simulink model "building3s"  (R2017a)
settings: Solver=ode14x  StartTime=0.0  StopTime=5  FixedStep=0.01  RelTol=1e-3
InitFcn:
  | kpmin=100;
  | kpmax=700;
  | kdmin=50;
  | kdmax=400;
values from neighbouring files (symbols this model uses):
  a = 175/98.3    (= 1.78026449644)    [Untitled.m]
  b = 50/98.3    (= 0.508646998983)    [Untitled.m]
  c = 1200000/98.3    (= 12207.5279756)    [Untitled.m]
  d = 684000/98.3    (= 6958.29094608)    [Untitled.m]
  e = 100/98.3    (= 1.01729399797)    [Untitled.m]
  f = 1370000/98.3    (= 13936.9277721)    [Untitled.m]
  jerm = 98.3    [Untitled.m]
  kkd = 253.2802    [Untitled.m]
  kki = 100    [Untitled.m]
  kkp = 570    [Untitled.m]
libraries: fuzblock x2, simulink x1
settings Model: Creator=Amir  LastModifiedBy=ASUS

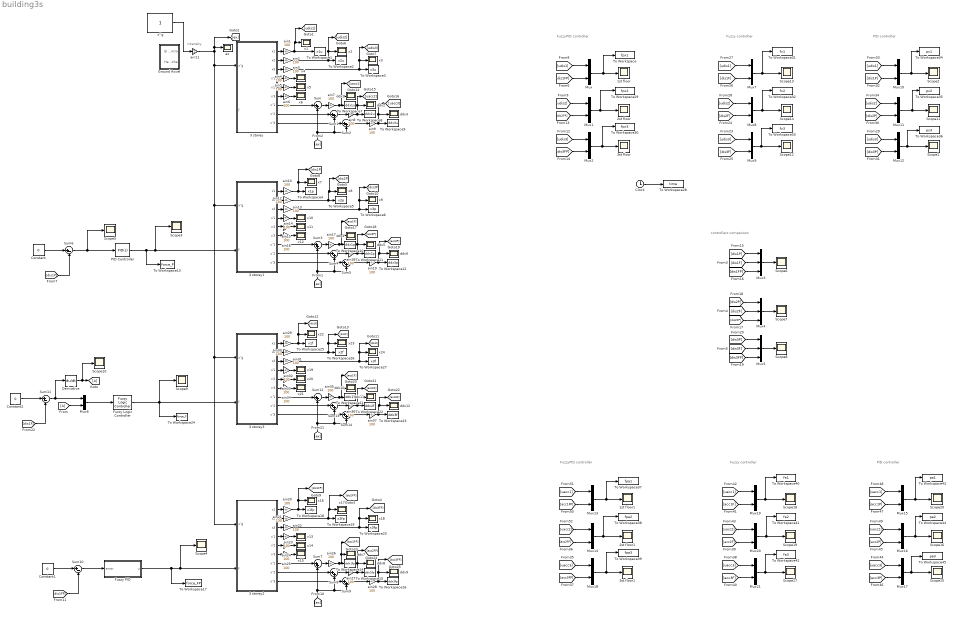
== system building3s ==
  note: controllers comparison
  note: Fuzzy controller
  note: FuzzyPID controller
  note: intensity
  note: PID controller
  note: Fuzzy controller
  note: FuzzyPID controller
  note: PID controller
  1st floor : Scope
  1st floor1 : Scope
  2st floor : Scope
  2st floor1 : Scope
  3 storey : Subsystem
  3 storey1 : Subsystem
  3 storey2 : Subsystem
  3 storey3 : Subsystem
  3st floor : Scope
  3st floor1 : Scope
  Clock : Clock
  Constant : Constant  Value=0
  Constant1 : Constant  Value=0
  Constant2 : Constant  Value=0
  Derivative : Derivative
  Fuzzy Logic Controller : fuzblock/Fuzzy Logic  Controller  fis=fuzz1
  Fuzzy PID : Subsystem
  Ground Accel : Subsystem
  Mux{,1..2,6..21} (19 alike) : Mux  Inputs=2
  Mux3 : Mux  Inputs=3
  Mux4 : Mux  Inputs=3
  Mux5 : Mux  Inputs=3
  PID Controller : simulink/Continuous/PID Controller  Controller=PID  TimeDomain=Continuous-time  SampleTime=-1  IntegratorMethod=Forward Euler  FilterMethod=Forward Euler  Form=Parallel  UseFilter=on  ControllerParametersSource=internal  P=kkp  I=kki  D=kkd  N=100  InitialConditionSource=internal  InitialConditionForIntegrator=0  InitialConditionForFilter=0  ExternalReset=none  LimitOutput=off  UpperSaturationLimit=inf  LowerSaturationLimit=-inf  LinearizeAsGain=on  AntiWindupMode=none  Kb=1  TrackingMode=off  Kt=1  PParamMin=[]  PParamMax=[]  IParamMin=[]  IParamMax=[]  DParamMin=[]  DParamMax=[]  NParamMin=[]  NParamMax=[]  KbParamMin=[]  KbParamMax=[]  KtParamMin=[]  KtParamMax=[]  POutMin=[]  POutMax=[]  IOutMin=[]  IOutMax=[]  DOutMin=[]  DOutMax=[]  NOutMin=[]  NOutMax=[]  KbOutMin=[]  KbOutMax=[]  KtOutMin=[]  KtOutMax=[]  IntegratorOutMin=[]  IntegratorOutMax=[]  FilterOutMin=[]  FilterOutMax=[]  SumOutMin=[]  SumOutMax=[]  SumI1OutMin=[]  SumI1OutMax=[]  SumI2OutMin=[]  SumI2OutMax=[]  SumI3OutMin=[]  SumI3OutMax=[]  SumDOutMin=[]  SumDOutMax=[]  SaturationOutMin=[]  SaturationOutMax=[]  IntegratorContinuousStateAttributes=''  IntegratorStateMustResolveToSignalObject=off  IntegratorRTWStateStorageClass=Auto  FilterContinuousStateAttributes=''  FilterStateMustResolveToSignalObject=off  FilterRTWStateStorageClass=Auto  DifferentiatorICPrevScaledInput=0  DifferentiatorOutMin=[]  DifferentiatorOutMax=[]  InitialConditionSetting=State (most efficient)
  Scope{1..20} (20 alike) : Scope
  Sum{,1..5,7..9,12..14} (12 alike) : Sum  Inputs=|++
  Sum10 : Sum  Inputs=|+-
  Sum11 : Sum  Inputs=|+-
  Sum6 : Sum  Inputs=|+-
  To Workspace : ToWorkspace  VariableName=fpx1  SampleTime=-1
  To Workspace1 : ToWorkspace  VariableName=x1u  SampleTime=-1
  To Workspace10 : ToWorkspace  VariableName=ddx1p  SampleTime=-1
  To Workspace11 : ToWorkspace  VariableName=ddx2p  SampleTime=-1
  To Workspace12 : ToWorkspace  VariableName=ddx3p  SampleTime=-1
  To Workspace13 : ToWorkspace  VariableName=force_P  SampleTime=-1
  To Workspace14 : ToWorkspace  VariableName=ddx1fp  SampleTime=-1
  To Workspace15 : ToWorkspace  VariableName=ddx2fp  SampleTime=-1
  To Workspace16 : ToWorkspace  VariableName=ddx3fp  SampleTime=-1
  To Workspace17 : ToWorkspace  VariableName=force_FP  SampleTime=-1
  To Workspace18 : ToWorkspace  VariableName=x1fp  SampleTime=-1
  To Workspace19 : ToWorkspace  VariableName=x2fp  SampleTime=-1
  To Workspace2 : ToWorkspace  VariableName=x2u  SampleTime=-1
  To Workspace20 : ToWorkspace  VariableName=x3fp  SampleTime=-1
  To Workspace21 : ToWorkspace  VariableName=ddx1f  SampleTime=-1
  To Workspace22 : ToWorkspace  VariableName=ddx2f  SampleTime=-1
  To Workspace23 : ToWorkspace  VariableName=ddx3f  SampleTime=-1
  To Workspace24 : ToWorkspace  VariableName=force_F  SampleTime=-1
  To Workspace25 : ToWorkspace  VariableName=x1f  SampleTime=-1
  To Workspace26 : ToWorkspace  VariableName=x2f  SampleTime=-1
  To Workspace27 : ToWorkspace  VariableName=x3f  SampleTime=-1
  To Workspace28 : ToWorkspace  VariableName=time  SampleTime=-1
  To Workspace29 : ToWorkspace  VariableName=fpx2  SampleTime=-1
  To Workspace3 : ToWorkspace  VariableName=x3u  SampleTime=-1
  To Workspace30 : ToWorkspace  VariableName=fpx3  SampleTime=-1
  To Workspace31 : ToWorkspace  VariableName=fx1  SampleTime=-1
  To Workspace32 : ToWorkspace  VariableName=fx2  SampleTime=-1
  To Workspace33 : ToWorkspace  VariableName=fx3  SampleTime=-1
  To Workspace34 : ToWorkspace  VariableName=px1  SampleTime=-1
  To Workspace35 : ToWorkspace  VariableName=px2  SampleTime=-1
  To Workspace36 : ToWorkspace  VariableName=px3  SampleTime=-1
  To Workspace37 : ToWorkspace  VariableName=fpa1  SampleTime=-1
  To Workspace38 : ToWorkspace  VariableName=fpa2  SampleTime=-1
  To Workspace39 : ToWorkspace  VariableName=fpa3  SampleTime=-1
  To Workspace4 : ToWorkspace  VariableName=x1p  SampleTime=-1
  To Workspace40 : ToWorkspace  VariableName=fa1  SampleTime=-1
  To Workspace41 : ToWorkspace  VariableName=fa2  SampleTime=-1
  To Workspace42 : ToWorkspace  VariableName=fa3  SampleTime=-1
  To Workspace43 : ToWorkspace  VariableName=pa1  SampleTime=-1
  To Workspace44 : ToWorkspace  VariableName=pa2  SampleTime=-1
  To Workspace45 : ToWorkspace  VariableName=pa3  SampleTime=-1
  To Workspace5 : ToWorkspace  VariableName=x2p  SampleTime=-1
  To Workspace6 : ToWorkspace  VariableName=x3p  SampleTime=-1
  To Workspace7 : ToWorkspace  VariableName=ddx1u  SampleTime=-1
  To Workspace8 : ToWorkspace  VariableName=ddx2u  SampleTime=-1
  To Workspace9 : ToWorkspace  VariableName=ddx3u  SampleTime=-1
  ain{1..10,12..37} (36 alike) : Gain  Gain=100
  ain11 : Gain
  ddx{1..12} (12 alike) : Scope
  ex : Scope
  x''g : Constant
  x{1..24} (24 alike) : Scope
  wires:
  ain3/1 -> To Workspace3/1, [udis3], x3/1
  3 storey/8(x''2) -> Sum1/1
  Sum/1 -> ain7/1
  [ex] -> Sum/2, Sum1/2, Sum2/2
  3 storey/5(x'2) -> ain5/1
  Sum2/1 -> ain9/1
  3 storey/7(x''1) -> Sum/1
  3 storey/9(x''3) -> Sum2/1
  ain9/1 -> To Workspace9/1, [uacc3], ddx3/1
  Sum1/1 -> ain8/1
  ain4/1 -> x4/1
  3 storey/6(x'3) -> ain6/1
  3 storey/4(x'1) -> ain4/1
  ain2/1 -> To Workspace2/1, [udis2], x2/1
  ain5/1 -> x5/1
  ain6/1 -> x6/1
  3 storey/3(x3) -> ain3/1
  ain7/1 -> To Workspace7/1, [uacc1], ddx1/1
  3 storey/2(x2) -> ain2/1
  ain1/1 -> To Workspace1/1, [udis1], x1/1
  ain11/1 -> 3 storey1/1(x''g), 3 storey2/1(x''g), 3 storey3/1(x''g), 3 storey/1(x''g), [ex], ex/1
  ain8/1 -> To Workspace8/1, ddx2/1, [uacc2]
  3 storey/1(x1) -> ain1/1
  x''g/1 -> ain11/1
  ain25/1 -> x15/1
  Sum7/1 -> ain26/1
  Sum10/1 -> Fuzzy PID/1(error)
  Constant1/1 -> Sum10/1
  3 storey2/8(x''2) -> Sum8/1
  [dis1FP] -> Sum10/2
  3 storey2/5(x'2) -> ain24/1
  Fuzzy PID/1(u) -> To Workspace17/1, Scope4/1, 3 storey2/2(f)
  ain22/1 -> [dis3FP], x18/1, To Workspace20/1
  3 storey2/2(x2) -> ain21/1
  [ex] -> Sum9/2, Sum8/2, Sum7/2
  Sum9/1 -> ain28/1
  3 storey2/3(x3) -> ain22/1
  ain26/1 -> [acc1FP], ddx7/1, To Workspace14/1
  ain28/1 -> [acc3FP], ddx9/1, To Workspace16/1
  ain20/1 -> [dis1FP], x16/1, To Workspace18/1
  ain21/1 -> [dis2FP], x17/1, To Workspace19/1
  Sum8/1 -> ain27/1
  3 storey2/6(x'3) -> ain25/1
  ain24/1 -> x14/1
  3 storey2/7(x''1) -> Sum7/1
  3 storey2/4(x'1) -> ain23/1
  3 storey2/1(x1) -> ain20/1
  3 storey2/9(x''3) -> Sum9/1
  ain23/1 -> x13/1
  ain27/1 -> [acc2FP], ddx8/1, To Workspace15/1
  3 storey1/8(x''2) -> Sum4/1
  ain14/1 -> x10/1
  3 storey1/1(x1) -> ain10/1
  ain10/1 -> [dis1P], x7/1, To Workspace4/1
  Sum3/1 -> ain17/1
  ain12/1 -> [dis2P], x8/1, To Workspace5/1
  ain19/1 -> [acc3P], ddx6/1, To Workspace12/1
  3 storey1/4(x'1) -> ain14/1
  ain17/1 -> [acc1P], ddx4/1, To Workspace10/1
  PID Controller/1 -> To Workspace13/1, Scope3/1, 3 storey1/2(f)
  Sum4/1 -> ain18/1
  ain18/1 -> [acc2P], ddx5/1, To Workspace11/1
  [ex] -> Sum5/2, Sum4/2, Sum3/2
  Sum5/1 -> ain19/1
  [dis1P] -> Sum6/2
  3 storey1/2(x2) -> ain12/1
  ain15/1 -> x11/1
  3 storey1/7(x''1) -> Sum3/1
  Constant/1 -> Sum6/1
  ain16/1 -> x12/1
  3 storey1/9(x''3) -> Sum5/1
  3 storey1/5(x'2) -> ain15/1
  ain13/1 -> [dis3P], x9/1, To Workspace6/1
  3 storey1/3(x3) -> ain13/1
  3 storey1/6(x'3) -> ain16/1
  Sum6/1 -> Scope5/1, PID Controller/1
  Mux5/1 -> Scope8/1
  Mux4/1 -> Scope7/1
  Mux3/1 -> Scope6/1
  [dis1FP] -> Mux3/3
  [dis1P] -> Mux3/1
  [dis2FP] -> Mux4/3
  [dis2P] -> Mux4/1
  [dis3P] -> Mux5/1
  [dis3FP] -> Mux5/3
  3 storey3/5(x'2) -> ain33/1
  ain36/1 -> ddx11/1, [acc2F], To Workspace22/1
  3 storey3/9(x''3) -> Sum14/1
  Constant2/1 -> Sum11/1
  ain30/1 -> [dis2F], x23/1, To Workspace26/1
  Derivative/1 -> Scope10/1, [A]
  [A] -> Mux6/2
  [ex] -> Sum14/2, Sum13/2, Sum12/2
  ain32/1 -> x19/1
  ain33/1 -> x20/1
  ain31/1 -> [dis3F], x24/1, To Workspace27/1
  Fuzzy Logic Controller/1 -> Scope9/1, 3 storey3/2(f), To Workspace24/1
  3 storey3/8(x''2) -> Sum13/1
  ain35/1 -> [acc1F], ddx10/1, To Workspace21/1
  Sum11/1 -> Derivative/1, Mux6/1
  ain34/1 -> x21/1
  Mux6/1 -> Fuzzy Logic Controller/1
  3 storey3/1(x1) -> ain29/1
  3 storey3/7(x''1) -> Sum12/1
  3 storey3/4(x'1) -> ain32/1
  3 storey3/3(x3) -> ain31/1
  Sum14/1 -> ain37/1
  3 storey3/2(x2) -> ain30/1
  ain37/1 -> [acc3F], ddx12/1, To Workspace23/1
  Sum13/1 -> ain36/1
  3 storey3/6(x'3) -> ain34/1
  [dis1F] -> Sum11/2
  Sum12/1 -> ain35/1
  ain29/1 -> [dis1F], x22/1, To Workspace25/1
  [dis2F] -> Mux4/2
  [dis1F] -> Mux3/2
  [dis3F] -> Mux5/2
  Mux1/1 -> To Workspace29/1, 2st floor/1
  Mux/1 -> To Workspace/1, 1st floor/1
  Mux2/1 -> To Workspace30/1, 3st floor/1
  [udis3] -> Mux2/1
  [udis2] -> Mux1/1
  [dis3FP] -> Mux2/2
  [dis2FP] -> Mux1/2
  [dis1FP] -> Mux/2
  [udis1] -> Mux/1
  [udis3] -> Mux9/1
  [dis1F] -> Mux7/2
  [dis2F] -> Mux8/2
  [udis1] -> Mux7/1
  Mux8/1 -> To Workspace32/1, Scope14/1
  [dis3F] -> Mux9/2
  Mux7/1 -> To Workspace31/1, Scope13/1
  Mux9/1 -> To Workspace33/1, Scope12/1
  [udis2] -> Mux8/1
  Mux12/1 -> To Workspace36/1, Scope1/1
  Mux10/1 -> To Workspace34/1, Scope2/1
  [udis3] -> Mux12/1
  [udis2] -> Mux11/1
  [udis1] -> Mux10/1
  Mux11/1 -> To Workspace35/1, Scope11/1
  [dis1P] -> Mux10/2
  [dis3P] -> Mux12/2
  [dis2P] -> Mux11/2
  Clock/1 -> To Workspace28/1
  [acc2P] -> Mux16/2
  [acc3P] -> Mux17/2
  [acc1P] -> Mux15/2
  Mux16/1 -> Scope16/1, To Workspace44/1
  [uacc1] -> Mux15/1
  [uacc2] -> Mux16/1
  [uacc3] -> Mux17/1
  Mux15/1 -> Scope20/1, To Workspace43/1
  Mux17/1 -> Scope15/1, To Workspace45/1
  [uacc2] -> Mux20/1
  Mux21/1 -> Scope17/1, To Workspace42/1
  Mux19/1 -> Scope18/1, To Workspace40/1
  [acc3F] -> Mux21/2
  Mux20/1 -> Scope19/1, To Workspace41/1
  [uacc1] -> Mux19/1
  [acc2F] -> Mux20/2
  [acc1F] -> Mux19/2
  [uacc3] -> Mux21/1
  [uacc1] -> Mux13/1
  [acc1FP] -> Mux13/2
  [acc2FP] -> Mux14/2
  [acc3FP] -> Mux18/2
  [uacc2] -> Mux14/1
  [uacc3] -> Mux18/1
  Mux18/1 -> 3st floor1/1, To Workspace39/1
  Mux13/1 -> 1st floor1/1, To Workspace37/1
  Mux14/1 -> 2st floor1/1, To Workspace38/1

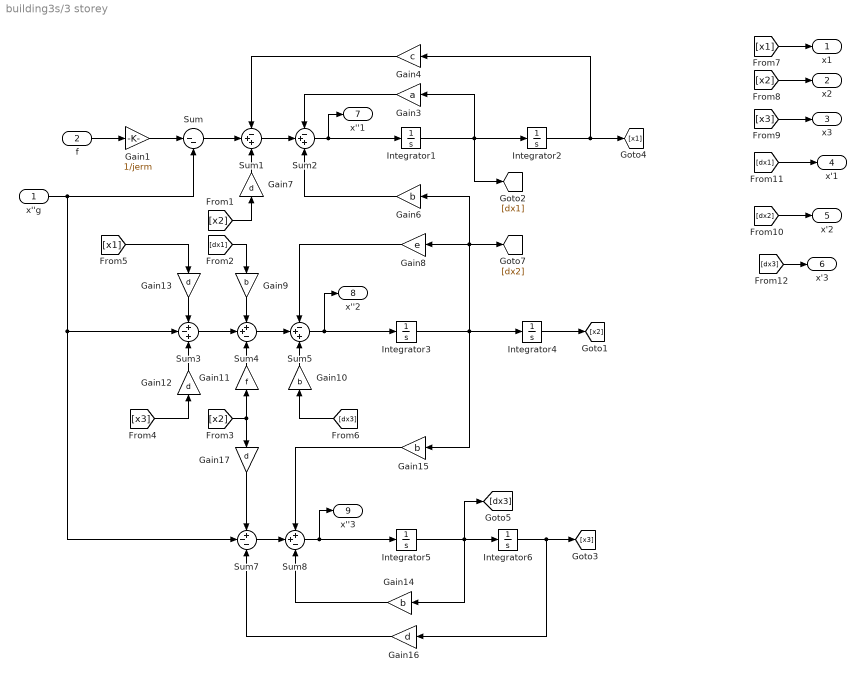
== system building3s/3 storey ==
  x''g : Inport
  f : Inport  Port=2
  Gain1 : Gain  Gain=1/jerm
  Gain{6,9..10,14..15} (5 alike) : Gain  Gain=b
  Gain11 : Gain  Gain=f
  Gain{7,12..13,16..17} (5 alike) : Gain  Gain=d
  Gain3 : Gain  Gain=a
  Gain4 : Gain  Gain=c
  Gain8 : Gain  Gain=e
  Integrator{1..6} (6 alike) : Integrator
  Sum : Sum  Inputs=|--
  Sum1 : Sum  Inputs=-++
  Sum2 : Sum  Inputs=-++
  Sum3 : Sum  Inputs=+-+
  Sum4 : Sum  Inputs=++-
  Sum5 : Sum  Inputs=-++
  Sum7 : Sum  Inputs=+--
  Sum8 : Sum  Inputs=++-
  x1 : Outport
  x2 : Outport  Port=2
  x3 : Outport  Port=3
  x'1 : Outport  Port=4
  x'2 : Outport  Port=5
  x'3 : Outport  Port=6
  x''1 : Outport  Port=7
  x''2 : Outport  Port=8
  x''3 : Outport  Port=9
  wires:
  Sum/1 -> Sum1/2
  Sum2/1 -> Integrator1/1, x''1/1
  Integrator1/1 -> Integrator2/1, Gain3/1, [dx1]
  f/1 -> Gain1/1
  Gain1/1 -> Sum/1
  Sum1/1 -> Sum2/2
  Sum3/1 -> Sum4/2
  Sum5/1 -> Integrator3/1, x''2/1
  Integrator3/1 -> Integrator4/1, Gain8/1, [dx2], Gain6/1, Gain15/1
  Sum4/1 -> Sum5/2
  Sum8/1 -> Integrator5/1, x''3/1
  Integrator5/1 -> Integrator6/1, Gain14/1, [dx3]
  Sum7/1 -> Sum8/2
  Gain3/1 -> Sum2/1
  Integrator2/1 -> Gain4/1, [x1]
  Gain4/1 -> Sum1/1
  Gain6/1 -> Sum2/3
  Integrator4/1 -> [x2]
  [x2] -> Gain7/1
  Gain7/1 -> Sum1/3
  x''g/1 -> Sum/2, Sum3/2, Sum7/2
  Gain8/1 -> Sum5/1
  [dx1] -> Gain9/1
  Gain9/1 -> Sum4/1
  [x2] -> Gain11/1, Gain17/1
  Gain11/1 -> Sum4/3
  Integrator6/1 -> [x3], Gain16/1
  [x3] -> Gain12/1
  Gain12/1 -> Sum3/3
  [x1] -> Gain13/1
  Gain13/1 -> Sum3/1
  Gain14/1 -> Sum8/3
  Gain16/1 -> Sum7/3
  [dx3] -> Gain10/1
  Gain10/1 -> Sum5/3
  [x1] -> x1/1
  [x2] -> x2/1
  [x3] -> x3/1
  [dx1] -> x'1/1
  [dx2] -> x'2/1
  [dx3] -> x'3/1
  Gain17/1 -> Sum7/1
  Gain15/1 -> Sum8/1

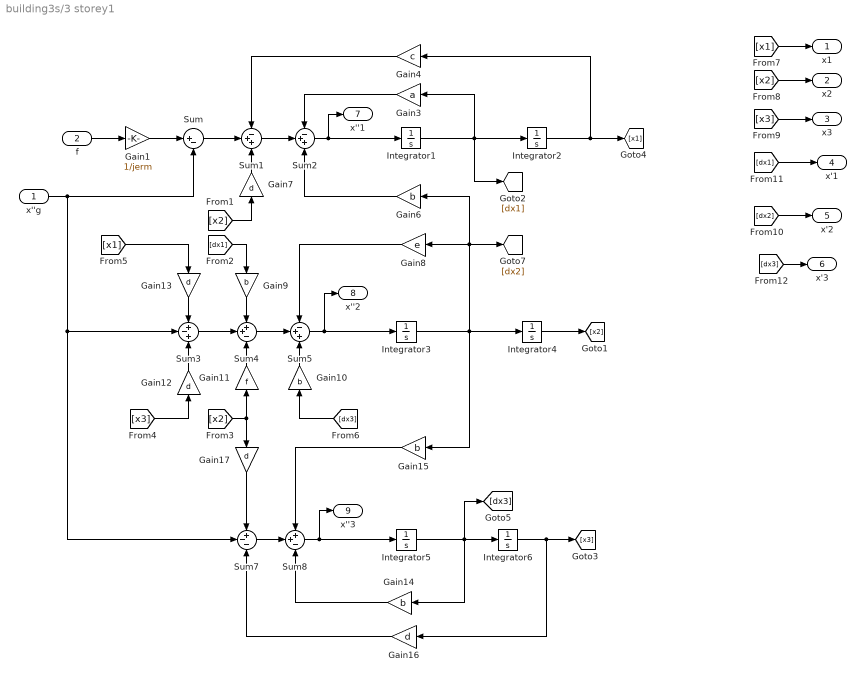
== system building3s/3 storey1 ==
  x''g : Inport
  f : Inport  Port=2
  Gain1 : Gain  Gain=1/jerm
  Gain{6,9..10,14..15} (5 alike) : Gain  Gain=b
  Gain11 : Gain  Gain=f
  Gain{7,12..13,16..17} (5 alike) : Gain  Gain=d
  Gain3 : Gain  Gain=a
  Gain4 : Gain  Gain=c
  Gain8 : Gain  Gain=e
  Integrator{1..6} (6 alike) : Integrator
  Sum : Sum  Inputs=|+-
  Sum1 : Sum  Inputs=-++
  Sum2 : Sum  Inputs=-++
  Sum3 : Sum  Inputs=+-+
  Sum4 : Sum  Inputs=++-
  Sum5 : Sum  Inputs=-++
  Sum7 : Sum  Inputs=+--
  Sum8 : Sum  Inputs=++-
  x1 : Outport
  x2 : Outport  Port=2
  x3 : Outport  Port=3
  x'1 : Outport  Port=4
  x'2 : Outport  Port=5
  x'3 : Outport  Port=6
  x''1 : Outport  Port=7
  x''2 : Outport  Port=8
  x''3 : Outport  Port=9
  wires:
  Gain15/1 -> Sum8/1
  Gain17/1 -> Sum7/1
  [dx3] -> x'3/1
  [dx2] -> x'2/1
  [dx1] -> x'1/1
  [x3] -> x3/1
  [x2] -> x2/1
  [x1] -> x1/1
  Gain10/1 -> Sum5/3
  [dx3] -> Gain10/1
  Gain16/1 -> Sum7/3
  Gain14/1 -> Sum8/3
  Gain13/1 -> Sum3/1
  [x1] -> Gain13/1
  Gain12/1 -> Sum3/3
  [x3] -> Gain12/1
  Integrator6/1 -> Gain16/1, [x3]
  Gain11/1 -> Sum4/3
  [x2] -> Gain17/1, Gain11/1
  Gain9/1 -> Sum4/1
  [dx1] -> Gain9/1
  Gain8/1 -> Sum5/1
  x''g/1 -> Sum7/2, Sum3/2, Sum/2
  Gain7/1 -> Sum1/3
  [x2] -> Gain7/1
  Integrator4/1 -> [x2]
  Gain6/1 -> Sum2/3
  Gain4/1 -> Sum1/1
  Integrator2/1 -> [x1], Gain4/1
  Gain3/1 -> Sum2/1
  Sum7/1 -> Sum8/2
  Integrator5/1 -> [dx3], Gain14/1, Integrator6/1
  Sum8/1 -> x''3/1, Integrator5/1
  Sum4/1 -> Sum5/2
  Integrator3/1 -> Gain15/1, Gain6/1, [dx2], Gain8/1, Integrator4/1
  Sum5/1 -> x''2/1, Integrator3/1
  Sum3/1 -> Sum4/2
  Sum1/1 -> Sum2/2
  Gain1/1 -> Sum/1
  f/1 -> Gain1/1
  Integrator1/1 -> [dx1], Gain3/1, Integrator2/1
  Sum2/1 -> x''1/1, Integrator1/1
  Sum/1 -> Sum1/2

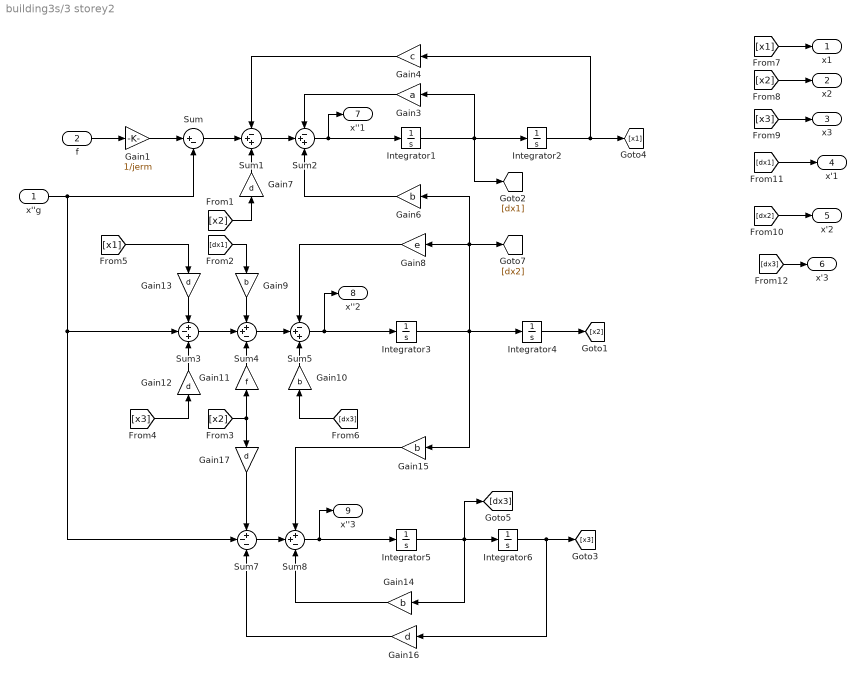
== system building3s/3 storey2 ==
  x''g : Inport
  f : Inport  Port=2
  Gain1 : Gain  Gain=1/jerm
  Gain{6,9..10,14..15} (5 alike) : Gain  Gain=b
  Gain11 : Gain  Gain=f
  Gain{7,12..13,16..17} (5 alike) : Gain  Gain=d
  Gain3 : Gain  Gain=a
  Gain4 : Gain  Gain=c
  Gain8 : Gain  Gain=e
  Integrator{1..6} (6 alike) : Integrator
  Sum : Sum  Inputs=|+-
  Sum1 : Sum  Inputs=-++
  Sum2 : Sum  Inputs=-++
  Sum3 : Sum  Inputs=+-+
  Sum4 : Sum  Inputs=++-
  Sum5 : Sum  Inputs=-++
  Sum7 : Sum  Inputs=+--
  Sum8 : Sum  Inputs=++-
  x1 : Outport
  x2 : Outport  Port=2
  x3 : Outport  Port=3
  x'1 : Outport  Port=4
  x'2 : Outport  Port=5
  x'3 : Outport  Port=6
  x''1 : Outport  Port=7
  x''2 : Outport  Port=8
  x''3 : Outport  Port=9
  wires:
  Gain15/1 -> Sum8/1
  Gain17/1 -> Sum7/1
  [dx3] -> x'3/1
  [dx2] -> x'2/1
  [dx1] -> x'1/1
  [x3] -> x3/1
  [x2] -> x2/1
  [x1] -> x1/1
  Gain10/1 -> Sum5/3
  [dx3] -> Gain10/1
  Gain16/1 -> Sum7/3
  Gain14/1 -> Sum8/3
  Gain13/1 -> Sum3/1
  [x1] -> Gain13/1
  Gain12/1 -> Sum3/3
  [x3] -> Gain12/1
  Integrator6/1 -> Gain16/1, [x3]
  Gain11/1 -> Sum4/3
  [x2] -> Gain17/1, Gain11/1
  Gain9/1 -> Sum4/1
  [dx1] -> Gain9/1
  Gain8/1 -> Sum5/1
  x''g/1 -> Sum7/2, Sum3/2, Sum/2
  Gain7/1 -> Sum1/3
  [x2] -> Gain7/1
  Integrator4/1 -> [x2]
  Gain6/1 -> Sum2/3
  Gain4/1 -> Sum1/1
  Integrator2/1 -> [x1], Gain4/1
  Gain3/1 -> Sum2/1
  Sum7/1 -> Sum8/2
  Integrator5/1 -> [dx3], Gain14/1, Integrator6/1
  Sum8/1 -> x''3/1, Integrator5/1
  Sum4/1 -> Sum5/2
  Integrator3/1 -> Gain15/1, Gain6/1, [dx2], Gain8/1, Integrator4/1
  Sum5/1 -> x''2/1, Integrator3/1
  Sum3/1 -> Sum4/2
  Sum1/1 -> Sum2/2
  Gain1/1 -> Sum/1
  f/1 -> Gain1/1
  Integrator1/1 -> [dx1], Gain3/1, Integrator2/1
  Sum2/1 -> x''1/1, Integrator1/1
  Sum/1 -> Sum1/2

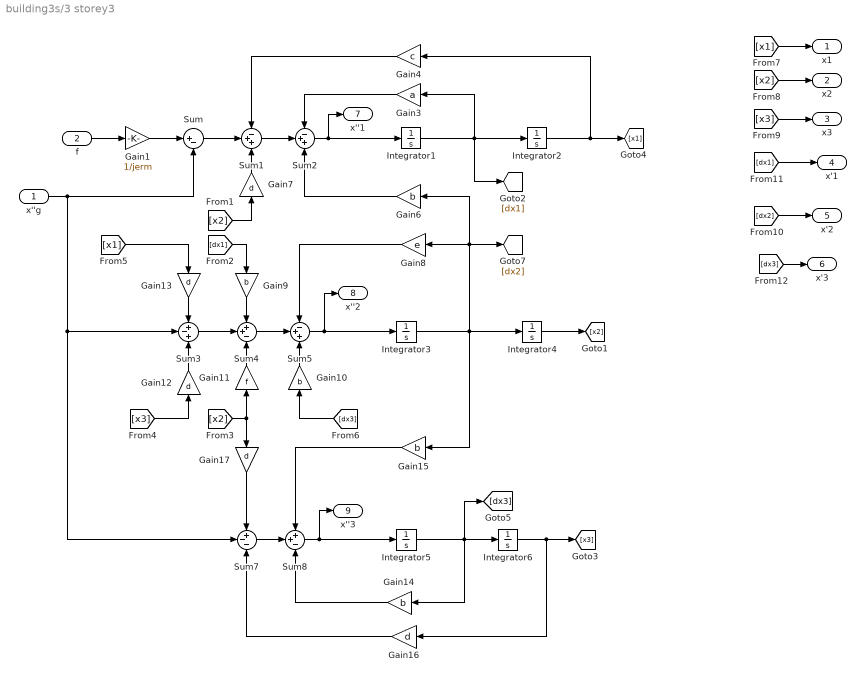
== system building3s/3 storey3 ==
  x''g : Inport
  f : Inport  Port=2
  Gain1 : Gain  Gain=1/jerm
  Gain{6,9..10,14..15} (5 alike) : Gain  Gain=b
  Gain11 : Gain  Gain=f
  Gain{7,12..13,16..17} (5 alike) : Gain  Gain=d
  Gain3 : Gain  Gain=a
  Gain4 : Gain  Gain=c
  Gain8 : Gain  Gain=e
  Integrator{1..6} (6 alike) : Integrator
  Sum : Sum  Inputs=|+-
  Sum1 : Sum  Inputs=-++
  Sum2 : Sum  Inputs=-++
  Sum3 : Sum  Inputs=+-+
  Sum4 : Sum  Inputs=++-
  Sum5 : Sum  Inputs=-++
  Sum7 : Sum  Inputs=+--
  Sum8 : Sum  Inputs=++-
  x1 : Outport
  x2 : Outport  Port=2
  x3 : Outport  Port=3
  x'1 : Outport  Port=4
  x'2 : Outport  Port=5
  x'3 : Outport  Port=6
  x''1 : Outport  Port=7
  x''2 : Outport  Port=8
  x''3 : Outport  Port=9
  wires:
  Gain15/1 -> Sum8/1
  Gain17/1 -> Sum7/1
  [dx3] -> x'3/1
  [dx2] -> x'2/1
  [dx1] -> x'1/1
  [x3] -> x3/1
  [x2] -> x2/1
  [x1] -> x1/1
  Gain10/1 -> Sum5/3
  [dx3] -> Gain10/1
  Gain16/1 -> Sum7/3
  Gain14/1 -> Sum8/3
  Gain13/1 -> Sum3/1
  [x1] -> Gain13/1
  Gain12/1 -> Sum3/3
  [x3] -> Gain12/1
  Integrator6/1 -> Gain16/1, [x3]
  Gain11/1 -> Sum4/3
  [x2] -> Gain17/1, Gain11/1
  Gain9/1 -> Sum4/1
  [dx1] -> Gain9/1
  Gain8/1 -> Sum5/1
  x''g/1 -> Sum7/2, Sum3/2, Sum/2
  Gain7/1 -> Sum1/3
  [x2] -> Gain7/1
  Integrator4/1 -> [x2]
  Gain6/1 -> Sum2/3
  Gain4/1 -> Sum1/1
  Integrator2/1 -> [x1], Gain4/1
  Gain3/1 -> Sum2/1
  Sum7/1 -> Sum8/2
  Integrator5/1 -> [dx3], Gain14/1, Integrator6/1
  Sum8/1 -> x''3/1, Integrator5/1
  Sum4/1 -> Sum5/2
  Integrator3/1 -> Gain15/1, Gain6/1, [dx2], Gain8/1, Integrator4/1
  Sum5/1 -> x''2/1, Integrator3/1
  Sum3/1 -> Sum4/2
  Sum1/1 -> Sum2/2
  Gain1/1 -> Sum/1
  f/1 -> Gain1/1
  Integrator1/1 -> [dx1], Gain3/1, Integrator2/1
  Sum2/1 -> x''1/1, Integrator1/1
  Sum/1 -> Sum1/2

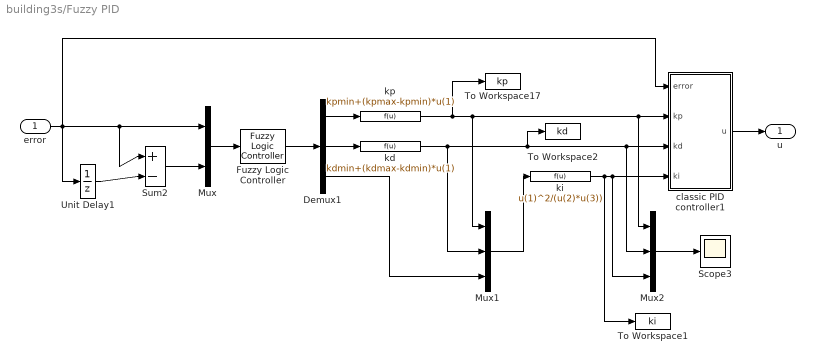
== system building3s/Fuzzy PID ==
  error : Inport
  Demux1 : Demux  Outputs=3
  Fuzzy Logic Controller : fuzblock/Fuzzy Logic  Controller  fis=FuzzyPID
  Mux : Mux  Inputs=2
  Mux1 : Mux  Inputs=3
  Mux2 : Mux  Inputs=3
  Scope3 : Scope
  Sum2 : Sum  Inputs=|+-
  To Workspace1 : ToWorkspace  VariableName=ki  SampleTime=-1
  To Workspace17 : ToWorkspace  VariableName=kp  SampleTime=-1
  To Workspace2 : ToWorkspace  VariableName=kd  SampleTime=-1
  Unit Delay1 : UnitDelay  SampleTime=-1
  classic PID controller1 : Subsystem
  kd : Fcn  Expr=kdmin+(kdmax-kdmin)*u(1)
  ki : Fcn  Expr=u(1)^2/(u(2)*u(3))
  kp : Fcn  Expr=kpmin+(kpmax-kpmin)*u(1)
  u : Outport
  wires:
  classic PID controller1/1(u) -> u/1
  error/1 -> Unit Delay1/1, Sum2/1, Mux/1, classic PID controller1/1(error)
  Unit Delay1/1 -> Sum2/2
  Sum2/1 -> Mux/2
  Mux/1 -> Fuzzy Logic Controller/1
  Fuzzy Logic Controller/1 -> Demux1/1
  Demux1/1 -> kp/1
  Demux1/2 -> kd/1
  Demux1/3 -> Mux1/3
  kp/1 -> To Workspace17/1, Mux1/1, Mux2/1, classic PID controller1/2(kp)
  kd/1 -> Mux1/2, To Workspace2/1, Mux2/2, classic PID controller1/3(kd)
  Mux1/1 -> ki/1
  ki/1 -> To Workspace1/1, Mux2/3, classic PID controller1/4(ki)
  Mux2/1 -> Scope3/1

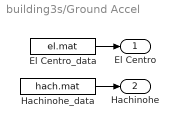
== system building3s/Ground Accel ==
  El Centro_data : FromFile  FileName=el.mat
  Hachinohe_data : FromFile  FileName=hach.mat
  El Centro : Outport
  Hachinohe : Outport  Port=2
  wires:
  El Centro_data/1 -> El Centro/1
  Hachinohe_data/1 -> Hachinohe/1

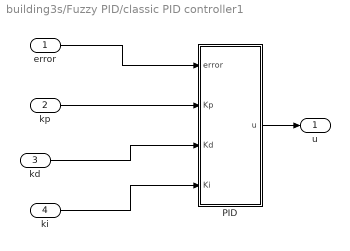
== system building3s/Fuzzy PID/classic PID controller1 ==
  error : Inport
  kp : Inport  Port=2
  kd : Inport  Port=3
  ki : Inport  Port=4
  PID : Subsystem
  u : Outport
  wires:
  PID/1(u) -> u/1
  ki/1 -> PID/4(Ki)
  kd/1 -> PID/3(Kd)
  kp/1 -> PID/2(Kp)
  error/1 -> PID/1(error)

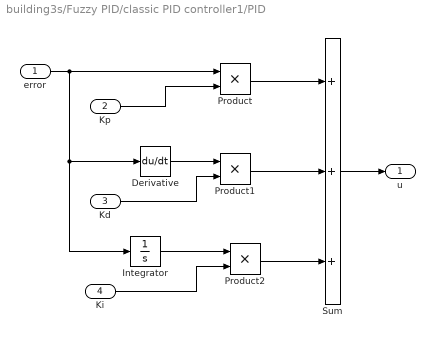
== system building3s/Fuzzy PID/classic PID controller1/PID ==
  error : Inport
  Kp : Inport  Port=2
  Kd : Inport  Port=3
  Ki : Inport  Port=4
  Derivative : Derivative
  Integrator : Integrator
  Product : Product
  Product1 : Product
  Product2 : Product
  Sum : Sum  Inputs=+++
  u : Outport
  wires:
  Sum/1 -> u/1
  Product2/1 -> Sum/3
  Product1/1 -> Sum/2
  Ki/1 -> Product2/2
  Integrator/1 -> Product2/1
  Kd/1 -> Product1/2
  Derivative/1 -> Product1/1
  Product/1 -> Sum/1
  Kp/1 -> Product/2
  error/1 -> Product/1, Derivative/1, Integrator/1
